simulink model "slexHARAndroidExample"  (R2021a)
settings: Solver=FixedStepAuto  StartTime=0.0  StopTime=10.0  RelTol=1e-3
model workspace (MAT data in the model file):
  jumpingImg = [255 255 255 255 255 255 255 255 255 255 255 255 ... (960000 elements, 800x400x3)]
  runningImg = [255 255 255 255 255 255 255 255 255 255 255 255 ... (960000 elements, 800x400x3)]
  sittingImg = [255 255 255 255 255 255 255 255 255 255 255 255 ... (960000 elements, 800x400x3)]
  standingImg = [255 255 255 255 255 255 255 255 255 255 255 255 ... (960000 elements, 800x400x3)]
  walkingImg = [255 255 255 255 255 255 255 255 255 255 255 255 ... (960000 elements, 800x400x3)]
undefined symbols (not defined in the file or in its folder): Acc_X, Acc_Y, Acc_Z, HARAndroidModel, Predicted_Activity
libraries: androiduilib x4, androidsensorlib x1, androidaudiovideolib x1
(part 2 of 2)

== system slexHARAndroidExample/More Info ==

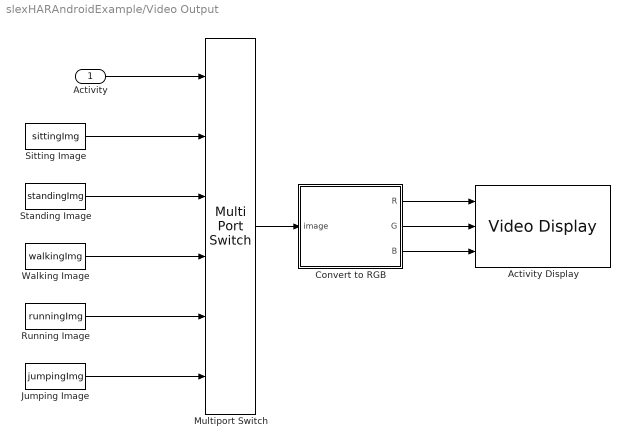
== system slexHARAndroidExample/Video Output ==
  Activity : Inport
  Activity Display : androidaudiovideolib/Video Display  BlockPlatform=Android
      settings: SourceProductBaseCode=ANDROID
  Convert to RGB : MATLAB Function  TreatAsAtomicUnit=on
  Jumping Image : Constant  Value=jumpingImg  VectorParams1D=off
  Multiport Switch : MultiPortSwitch  Inputs=5  DiagnosticForDefault=None
  Running Image : Constant  Value=runningImg  VectorParams1D=off
  Sitting Image : Constant  Value=sittingImg  VectorParams1D=off
  Standing Image : Constant  Value=standingImg  VectorParams1D=off
  Walking Image : Constant  Value=walkingImg  VectorParams1D=off
  wires:
  Convert to RGB/3(B) -> Activity Display/3
  Standing Image/1 -> Multiport Switch/3
  Jumping Image/1 -> Multiport Switch/6
  Activity/1 -> Multiport Switch/1
  Convert to RGB/1(R) -> Activity Display/1
  Multiport Switch/1 -> Convert to RGB/1(image)
  Convert to RGB/2(G) -> Activity Display/2
  Sitting Image/1 -> Multiport Switch/2
  Running Image/1 -> Multiport Switch/5
  Walking Image/1 -> Multiport Switch/4

== matlab function slexHARAndroidExample/Video Output/Convert to RGB ==
  data: image input; R output; G output; B output
function [R,G,B] = deconcatenate(image)
% deconcatenate - Extract Red, Green and Blue channels from a RGB image. 

% Copyright 2017 The MathWorks, Inc.

R = image(:,:,1);
G = image(:,:,2);
B = image(:,:,3);

== matlab function slexHARAndroidExample/extractFeatures ==
  data: xbuffer input single size=[32 1]; features output double size=[1 60]; ybuffer input single size=[32 1]; zbuffer input single size=[32 1]
%% extractFeatures extractFeatures from real-time accelerometer, 3 axes data 
% returns 1xk vector, where k is is the number of features (k = 60 for this
% problem)
% Copyright 2017 The MathWorks, Inc.

function features  = extractFeatures(xbuffer, ybuffer, zbuffer)

% set sample time and frequency 
sample_time = 0.1;
frequency   = (1/sample_time); 

% pre-computed fmean and fstd values from training data
acceleration = [xbuffer ybuffer zbuffer];

%% Extract features
features = featuresFromBuffer(acceleration, frequency);

end

function feature = featuresFromBuffer(at, fs)
% featuresFromBuffer Extract vector of features from raw data buffer
%
% feat1-3 = mean (3 axis);
% feat4-6 = rms (3);
% feat7-15 = autocorrelation: height of main peak; height and position of second peak (3 feature *3 axis);
% feat16-51 = Spectral peak features: height and position of first 6 peaks% (12 feature * 3 axis);
% feat51-60 = Spectral power features: total power in 5 adjacent and pre-defined frequency bands (5 feature * 3 axis);

% Initialize digital filter
persistent dcblock corr spect f
if(isempty(dcblock))
    [s,g] = getFilterCoefficients();
    dcblock = dsp.BiquadFilter('Structure','Direct form II transposed', ...
        'SOSMatrix',s,'ScaleValues',g);

    NFFT = 4096;
    spect = dsp.SpectrumEstimator('SpectralAverages',1,...
        'Window','Rectangular','FrequencyRange','onesided',...
        'SampleRate',fs,'SpectrumType','Power density',...
        'FFTLengthSource','Property','FFTLength',4096);
    f = (fs/NFFT)*(0:NFFT/2)';

    corr = dsp.Autocorrelator;
end

% Initialize feature vector
feature = zeros(1,60);

% Average value in signal buffer for all three acceleration components (1 each)
feature(1:3) = mean(at,1);

% Remove gravitational contributions with digital filter
ab = step(dcblock,at);

% RMS value in signal buffer for all three acceleration components (1 each)
feature(4:6) = rms(ab,1);

% Pre-compute spectra of 3 channels for frequency-domain features
af = step(spect,ab);

% Spectral peak features (12 per channel): value and freq of first 6 peaks
feature(16:51) = spectralPeaksFeatures(af, f);

% Spectral power features (5 each): total power in 5 adjacent
% and pre-defined frequency bands
feature(52:60) = spectralPowerFeatures(af, f);

% Autocorrelation features for all three acceleration components (3 each): 
% height of main peak; height and position of second peak
feature(7:15) = autocorrFeatures(ab, corr, fs);

end

%% ===== HELPER FUNCTIONS =====
% Calculate autocorrelation features: feat7-15
% height of main peak; height and position of second peak
function feats = autocorrFeatures(x, corr, fs)

feats = zeros(1,9);

c = step(corr, x);
lags = (0:length(x)-1)';

minprom = 0.0005;
mindist_xunits = 0.3;
minpkdist = floor(mindist_xunits/(1/fs));

% Separate peak analysis for 3 different channels
for k = 1:3
    [pks,locs] = findpeaks([0;c(:,k)],...
        'minpeakprominence',minprom,...
        'minpeakdistance',minpkdist);

    tc = (1/fs)*lags;
    tcl = tc(locs-1);

    % Feature 1 - peak height at 0
    feats(3*(k-1)+1) = c(1,k);
    % Features 2 and 3 - position and height of first peak 
    if(length(tcl) >= 2)   % else f2,f3 already 0
        feats(3*(k-1)+2) = tcl(2);
        feats(3*(k-1)+3) = pks(2);
    end
end
end

% Calculate spectral peak features: feat16-51 
% height and position of first 6 peaks
function feats = spectralPeaksFeatures(xpsd, f)

feats = zeros(1,3*12);

mindist_xunits = 0.3;
minpkdist = floor(mindist_xunits/f(2));

% iterate through number of channels
nfinalpeaks = 6;
for k = 1:3
    [pks,locs] = findpeaks(xpsd(:,k),'npeaks',20,'minpeakdistance',minpkdist);
    opks = typecast(zeros(nfinalpeaks,1), 'single');
    olocs = zeros(nfinalpeaks,1); 
    if(~isempty(pks))
        mx = min(6,length(pks));
        [spks, idx] = sort(pks,'descend');
        slocs = locs(idx);

        pkssel = spks(1:mx);
        locssel = slocs(1:mx);

        [olocs, idx] = sort(locssel,'ascend');
        opks = pkssel(idx);
    end
    ofpk = f(olocs);

    % Features 1-6 positions of highest 6 peaks
    feats(12*(k-1)+(1:length(opks))) = ofpk;
    % Features 7-12 power levels of highest 6 peaks
    feats(12*(k-1)+(7:7+length(opks)-1)) = opks;
end
end

% Calculate spectral power features: feat51-60 
% total power in 5 adjacent and pre-defined frequency bands (5 feature * 3 axis);
function feats = spectralPowerFeatures(xpsd, f)

edges = [0.5, 5, 10, 20];
featstmp = zeros(3,3);
    
for kband = 1:length(edges)-1
    featstmp(kband,:) = sum(xpsd( (f>=edges(kband)) & (f<edges(kband+1)), : ),1);
end
feats = featstmp(:);
end

function [s,g] = getFilterCoefficients()
    coder.extrinsic('zp2sos')
    [z,p,k] = ellip(7,0.1,60,0.4/25,'high');
    [s,g] = coder.const(@zp2sos,z,p,k);
end

== matlab function slexHARAndroidExample/calibrate ==
  data: x input single size=[1 1]; xout output size=[1 1]; y input single size=[1 1]; z input single size=[1 1]; yout output; zout output
function [xout,yout,zout] = calibrate(x,y,z)%#codegen
% calibrate - Static calibration of the accelerometer for an
% Android device. 

% Copyright 2017 The MathWorks, Inc.

calibrationstr = coder.load('slexHARAndroidCalibrationMatrix.mat');
calibrationMatrix = coder.const(calibrationstr.AndroidCalibrationMatrix);

out = [x,y,z,1]*calibrationMatrix;
xout = out(1);
yout = out(2);
zout = out(3);

== matlab function slexHARAndroidExample/predictActivity ==
  data: u input; y output
function y = predictActivity(u)%#codegen
% predictActivity - predict human activity based on trained model stored in
%   EnsembleModelAndroid.mat file.

% Copyright 2017 The MathWorks, Inc.

persistent mdl;

if isempty(mdl)
   mdl = loadLearnerForCoder('EnsembleModel.mat'); 
end

y = predict(mdl,u);

end
